simulink model "od_stanu"  (R2023a)
settings: Solver=VariableStepAuto  StartTime=0.0  StopTime=10  RelTol=1e-3
values from neighbouring files (symbols this model uses):
  K = acker(A, B, [sb, sb, sb])    [do_workspace.m]    (also in zadania_1_5.m)
settings Model: Creator=adams  LastModifiedBy=adams

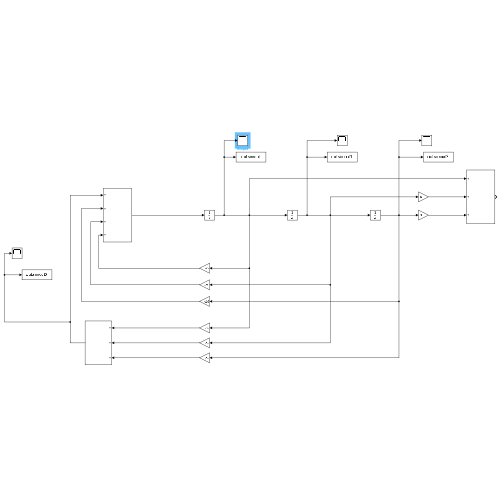
[thumbnail: Simulink's stored preview of the top-level diagram]
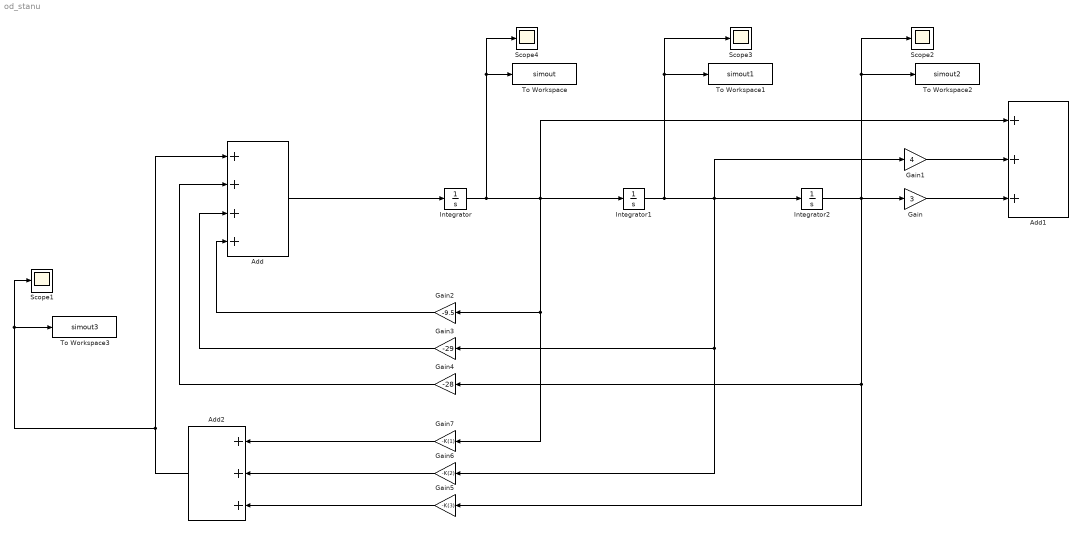
== system od_stanu ==
  Add : Sum  Inputs=++++
  Add1 : Sum  Inputs=+++
  Add2 : Sum  Inputs=+++
  Gain : Gain  Gain=3
  Gain1 : Gain  Gain=4
  Gain2 : Gain  Gain=-9.5
  Gain3 : Gain  Gain=-29
  Gain4 : Gain  Gain=-28
  Gain5 : Gain  Gain=-K(3)
  Gain6 : Gain  Gain=-K(2)
  Gain7 : Gain  Gain=-K(1)
  Integrator : Integrator  InitialCondition=-1
  Integrator1 : Integrator  InitialCondition=-1
  Integrator2 : Integrator  InitialCondition=2
  Scope{1..4} (4 alike) : Scope
  To Workspace : ToWorkspace  VariableName=simout  SaveFormat=Structure With Time  SampleTime=-1
  To Workspace1 : ToWorkspace  VariableName=simout1  SaveFormat=Structure With Time  SampleTime=-1
  To Workspace2 : ToWorkspace  VariableName=simout2  SaveFormat=Structure With Time  SampleTime=-1
  To Workspace3 : ToWorkspace  VariableName=simout3  SaveFormat=Structure With Time  SampleTime=-1
  wires:
  Integrator2/1 -> To Workspace2/1, Scope2/1, Gain5/1, Gain4/1, Gain/1
  Gain/1 -> Add1/3
  Integrator1/1 -> To Workspace1/1, Scope3/1, Integrator2/1, Gain6/1, Gain3/1, Gain1/1
  Gain1/1 -> Add1/2
  Integrator/1 -> To Workspace/1, Scope4/1, Gain7/1, Gain2/1, Add1/1, Integrator1/1
  Add/1 -> Integrator/1
  Gain2/1 -> Add/4
  Gain3/1 -> Add/3
  Gain4/1 -> Add/2
  Add2/1 -> To Workspace3/1, Scope1/1, Add/1
  Gain7/1 -> Add2/1
  Gain6/1 -> Add2/2
  Gain5/1 -> Add2/3
